simulink model "Stanley_Querregler"  (R2019b)
settings: Solver=FixedStepAuto  StartTime=0.0  StopTime=10.0  FixedStep=1e-2  RelTol=1e-3
libraries: robotlib x7, drivingvehiclecontroller x1

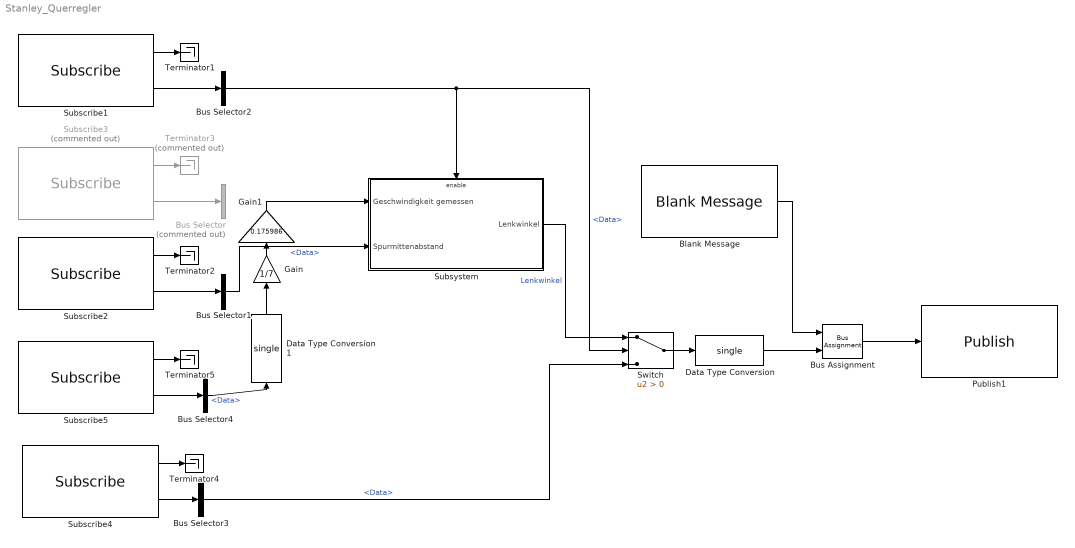
== system Stanley_Querregler ==
  Blank Message : robotlib/Blank Message  messageClass=Message  entityType=std_msgs/Float32  messageType=std_msgs/Float32  SampleTime=inf
  Bus Assignment : BusAssignment  AssignedSignals=Data
  Bus Selector : BusSelector  Commented=on  OutputSignals=Data
  Bus Selector{1..4} (4 alike) : BusSelector  OutputSignals=Data
  Data Type Conversion : DataTypeConversion  OutDataTypeStr=single
  Data Type Conversion1 : DataTypeConversion  OutDataTypeStr=single
  Gain : Gain  Gain=1/7
  Gain1 : Gain  Gain=0.175986
  Publish1 : robotlib/Publish  topicSource=Specify your own  topic=/ctl_servoAngle  messageType=std_msgs/Float32  messageQueueLength=1
  Subscribe1 : robotlib/Subscribe  topicSource=Specify your own  topic=/trj_enableLateralControl  messageType=std_msgs/Bool  sampleTime=-1  messageQueueLength=1
  Subscribe2 : robotlib/Subscribe  topicSource=Specify your own  topic=/trj_deltaY  messageType=std_msgs/Float32  sampleTime=-1  messageQueueLength=1
  Subscribe3 : robotlib/Subscribe  Commented=on  topicSource=Specify your own  topic=/ctl_velocity  messageType=std_msgs/Float32  sampleTime=-1  messageQueueLength=1
  Subscribe4 : robotlib/Subscribe  topicSource=Specify your own  topic=/trj_steeringAngle  messageType=std_msgs/Float32  sampleTime=-1  messageQueueLength=1
  Subscribe5 : robotlib/Subscribe  topicSource=Specify your own  topic=/ctl_motorRpm  messageType=std_msgs/Int16  sampleTime=-1  messageQueueLength=1
  Subsystem : Subsystem
  Switch : Switch  Criteria=u2 > Threshold
  Terminator{1..2,4..5} (4 alike) : Terminator
  Terminator3 : Terminator  Commented=on
  wires:
  Subscribe3/1 -> Terminator3/1
  Subscribe3/2 -> Bus Selector/1
  Subscribe2/2 -> Bus Selector1/1
  Subscribe2/1 -> Terminator2/1
  Bus Selector1/1 -> Subsystem/2(Spurmittenabstand)  "<Data>"
  Data Type Conversion/1 -> Bus Assignment/2
  Blank Message/1 -> Bus Assignment/1
  Bus Assignment/1 -> Publish1/1
  Subscribe1/1 -> Terminator1/1
  Subscribe1/2 -> Bus Selector2/1
  Bus Selector2/1 -> Subsystem/Enable, Switch/2  "<Data>"
  Subscribe4/1 -> Terminator4/1
  Subscribe4/2 -> Bus Selector3/1
  Bus Selector3/1 -> Switch/3  "<Data>"
  Subsystem/1(Lenkwinkel) -> Switch/1  "Lenkwinkel"
  Switch/1 -> Data Type Conversion/1
  Subscribe5/1 -> Terminator5/1
  Bus Selector4/1 -> Data Type Conversion1/1  "<Data>"
  Subscribe5/2 -> Bus Selector4/1
  Gain/1 -> Gain1/1
  Gain1/1 -> Subsystem/1(Geschwindigkeit gemessen)
  Data Type Conversion1/1 -> Gain/1

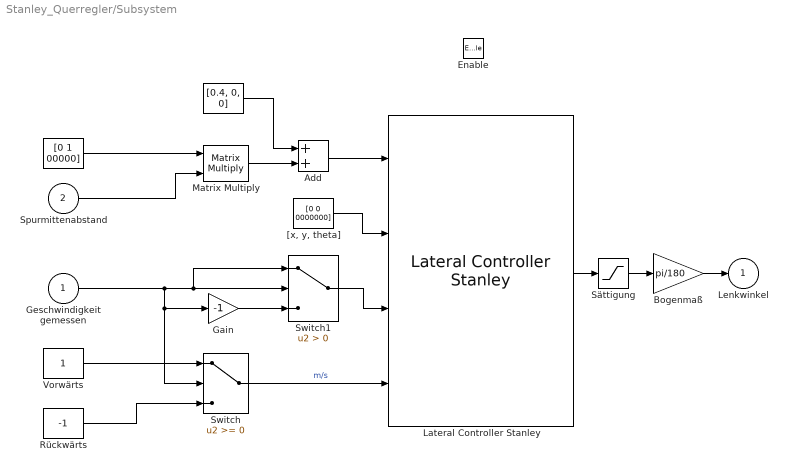
== system Stanley_Querregler/Subsystem ==
  Geschwindigkeit gemessen : Inport
  Spurmittenabstand : Inport  Port=2
  Enable : EnablePort
  " " : Constant  Value=[0.4, 0, 0]
  " " : Constant  Value=[0 1 00000]
  Add : Sum
  Bogenmaß : Gain  Gain=pi/180
  Gain : Gain  Gain=-1
  Lateral Controller Stanley : drivingvehiclecontroller/Lateral Controller Stanley  ModelType=Kinematic bicycle model  PositionGainF=2.5  PositionGainR=2.5  YawRateGain=0.2  DelayGain=0.2  VehicleMass=1575  Lf=1.2  Lr=1.6  TireStiffness=19000  Wheelbase=0.25  MaxSteeringAngle=20
  Matrix Multiply : Product  Multiplication=Matrix(*)
  Rückwärts : Constant  Value=-1
  Switch : Switch
  Switch1 : Switch  Criteria=u2 > Threshold
  Sättigung : Saturate  UpperLimit=20  LowerLimit=-20
  Vorwärts : Constant
  "[x, y, theta]" : Constant  Value=[0 0 0000000]
  Lenkwinkel : Outport
  wires:
  " "/1 -> Add/1
  Add/1 -> Lateral Controller Stanley/1
  Switch1/1 -> Lateral Controller Stanley/3
  Geschwindigkeit gemessen/1 -> Switch/2, Gain/1, Switch1/2, Switch1/1
  Sättigung/1 -> Bogenmaß/1
  Bogenmaß/1 -> Lenkwinkel/1
  Matrix Multiply/1 -> Add/2
  "[x, y, theta]"/1 -> Lateral Controller Stanley/2
  Spurmittenabstand/1 -> Matrix Multiply/2
  Rückwärts/1 -> Switch/3
  Vorwärts/1 -> Switch/1
  " "/1 -> Matrix Multiply/1
  Switch/1 -> Lateral Controller Stanley/4  "m/s"
  Gain/1 -> Switch1/3
  Lateral Controller Stanley/1 -> Sättigung/1
